simulink library "Airframes"  (Simulink 7.3)
settings: Solver=ode45  StartTime=0.0  StopTime=10.0  RelTol=1e-3
undefined symbols (not defined in the file or in its folder): Vo
libraries: aero_sim_lib x4, simulink x2
(part 1 of 2)
settings Model: Creator=Administrator  LastModifiedBy=Administrator

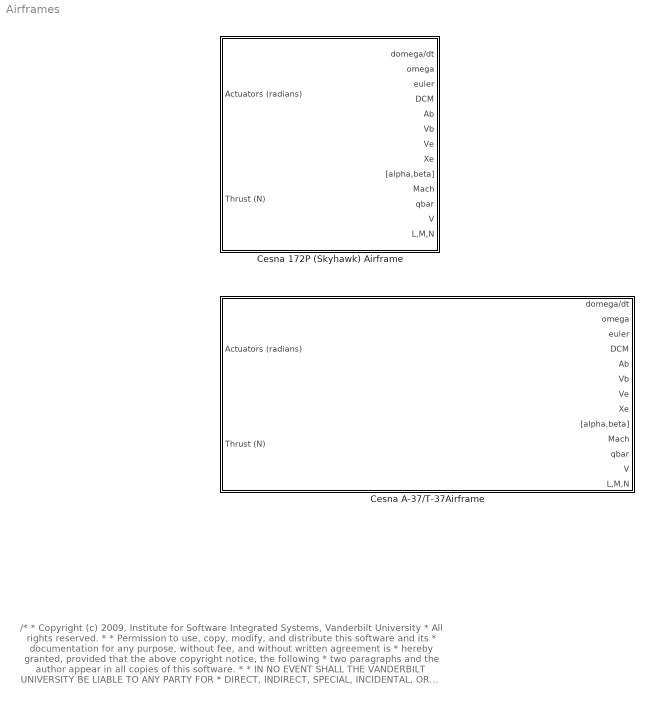
== system Airframes ==
  note: /*
      |  * Copyright (c) 2009, Institute for Software Integrated Systems, Vanderbilt University
      |  * All rights reserved.
      |  *
      |  * Permission to use, copy, modify, and distribute this software and its
      |  * documentation for any purpose, without fee, and without written agreement is
      |  * hereby granted, provided that the above copyright notice, the following
      |  * two paragraphs and the author appear in all copies of this software.
      |  *
      |  * IN NO EVENT SHALL THE VANDERBILT UNIVERSITY BE LIABLE TO ANY PARTY FOR
      |  * DIRECT, INDIRECT, SPECIAL, INCIDENTAL, OR CONSEQUENTIAL DAMAGES ARISING OUT
      |  * OF THE USE OF THIS SOFTWARE AND ITS DOCUMENTATION, EVEN IF THE VANDERBILT
      |  * UNIVERSITY HAS BEEN ADVISED OF THE POSSIBILITY OF SUCH DAMAGE.
      |  *
      |  * THE VANDERBILT UNIVERSITY SPECIFICALLY DISCLAIMS ANY WARRANTIES,
      |  * INCLUDING, BUT NOT LIMITED TO, THE IMPLIED WARRANTIES OF MERCHANTABILITY
      |  * AND FITNESS FOR A PARTICULAR PURPOSE.  THE SOFTWARE PROVIDED HEREUNDER IS
      |  * ON AN "AS IS" BASIS, AND THE VANDERBILT UNIVERSITY HAS NO OBLIGATION TO
      |  * PROVIDE MAINTENANCE, SUPPORT, UPDATES, ENHANCEMENTS, OR MODIFICATIONS.
      |  *
      |  * @author Nicholas Kottenstette
      |  */
  Cesna 172P (Skyhawk) Airframe : Subsystem  mask{trim_enable=off, XYZe_0=[0,0,-1000], V=Vo, Vb_0=Vo*[1,0,.0184], euler_0=[0,.018,0], omega_0=zeros(3,1), M=.4535959237*1043.3, I=[1285.3,0,0;0,1824.9,0;0,0,2666.9], b=10.9118, cbar=1.4935, S=16.1651, CG=[0,0,0], CP=[0,0,0], CD_p=[0.031,  0.13,  0,  0.06,  0], CL_p=[0.31,   5.143,    3.9,   0.43,   0], CY_p=[0,  -0.31,  -0.037,  0.21,  0.0,  0.187], Clm_p=[0, -0.089,  -0.47,  0.096,  -0.178,  0.0147], Cmm_p=[-0.015, -0.89,  -12.4,  -1.28,  0], Cnm_p=[0,  0.065, -0.03,  -0.099,  0.053,  -0.0657], delta_f=0, k_wind=off}
      mask prompts: trim_enable "Enable trim calculation"; XYZe_0 "Initial Inertial Position [XYZe_0] (meters)"; V "V (aero-velocity) (m/s)"; Vb_0 "Initial Body Velocity [Vb_0] (meters/sec)"; euler_0 "Initial Euler [euler_0] [roll,pitch,yaw] (radians)"; omega_0 "Initial Body Rotation Rates [omega_0] (rad/sec)"; M "Mass [M] (kg)"; I "Inertial Matrix [I] [Ixx,0,-Ixz;0,Iyy,0;-Ixz,0,Izz]"; b "Wing Span [b] (meters)"; cbar "MAC [cbar] (meters)"; S "Wing Area [S] (meters^2)"; CG "CG [CG] (meters)"; CP "CP [CP] (meters)"; CD_p "Drag Parameters:CD_p= [CD0,CDa,CDq,CDde,CDin]"; CL_p "Lift Parameters:CL_p=[CL0,CLa,CLq,CLde,CLin]"; CY_p "Y-Drag Parameters:CY_p=[CY0,CYb,CYp,CYr,CYda,CYdr]"; Clm_p "L-Moment (about-x_b) Parameters:Clm_p=[Cl0,Clb,Clp,Clr,Clda,Cldr]"; Cmm_p "M-Moment (about-y_b) Parameters:Cmm_p=[Cm0,Cma,Cmq,Cmde,Cmin]"; Cnm_p "N-Moment (about-z_b) Parameters:Cnm_p=[Cn0,Cnb,Cnp,Cnr,Cnda,Cndr]"; k_wind "wind dist on"
      mask init:
      | h=abs(XYZe_0(3));
      | if trim_enable
      |     [F_T_trim,alpha_trim,delta_e_trim,Sol] = fixed_wing_trim(CD_p,CL_p,Cmm_p,S,V,h,M,delta_f,[],false);
      |     u=V*sqrt(1/(1+tan(alpha_trim)^2));
      |     w=u*tan(alpha_trim);
      |     Vb_0=[u,0,w];
      |     euler_0(2)=alpha_trim;
      | end
      mask Display:
      | image(imread('Cessna_172P.jpg','jpg'))
      | color('black');port_label('output',1,'d\omega/dt','texmode','on')
      | port_label('output',2,'\omega','texmode','on')
      | port_label('output',3,'\eta^T=[\phi,\theta,\psi]^T','texmode','on')
      | port_label('output',4,'R(\eta)','texmode','on')
      | port_label('output',5,'A_b(m/s^2','texmode','on')
      | port_label('output',6,'V_b(m/s)','texmode','on')
      | port_label('output',7,'V_I(m/s)','texmode','on')
      | port_label('output',8,'X_I(m)','texmode','on')
      | port_label('output',9,'[\alpha,\beta]','texmode','on')
      | port_label('output',10,'Mach (V/a)')
      | port_label('output',11,'q_bar')
      | port_label('output',12,'V')
      | port_label('output',13,'L,M,N')
      | port_label('input',1,'[\delta_e,\delta_f,\delta_a,\delta_r](radians)','texmode','on')
      | port_label('input',2,'Thrust (N)')
  Cesna A-37/T-37Airframe : Subsystem  mask{trim_enable=off, XYZe_0=[0,0,-1000], V=Vo, Vb_0=Vo*[1,0,.0184], euler_0=[0,.018,0], omega_0=zeros(3,1), M=.4535959237*6360, I=1.35581795*[7.99e3,0,2.34e2;0,3.33e3,0;2.34e2,0,1.12e4], b=.3048*33.8, cbar=.3048*5.47, S=(.3048^2)*182, CG=[0,0,0], CP=[0,0,0], CD_p=[0.048,  0.384,  0,  0,  0], CL_p=[0.2,   5.15,    4.1,   0.5,   0], CY_p=[0,  -0.346,  -0.0827,  0.3,  0.0,  0.2], Clm_p=[0, -0.0944,  -0.442,  0.0926,  -0.181,  0.015], Cmm_p=[0.025, -0.7,  -14.9,  -1.12,  0], Cnm_p=[0,  0.1106, -0.0243,  -0.139,  0.0254,  -0.0365], delta_f=0, k_wind=off}
      mask prompts: trim_enable "Enable Trim Calculation"; XYZe_0 "Initial Inertial Position [XYZe_0] (meters)"; V "V (aero-velocity) (m/s)"; Vb_0 "Initial Body Velocity [Vb_0] (meters/sec)"; euler_0 "Initial Euler [euler_0] [roll,pitch,yaw] (radians)"; omega_0 "Initial Body Rotation Rates [omega_0] (rad/sec)"; M "Mass [M] (kg)"; I "Inertial Matrix [I] [Ixx,0,-Ixz;0,Iyy,0;-Ixz,0,Izz]"; b "Wing Span [b] (meters)"; cbar "MAC [cbar] (meters)"; S "Wing Area [S] (meters^2)"; CG "CG [CG] (meters)"; CP "CP [CP] (meters)"; CD_p "Drag Parameters:CD_p= [CD0,CDa,CDq,CDde,CDin]"; CL_p "Lift Parameters:CL_p=[CL0,CLa,CLq,CLde,CLin]"; CY_p "Y-Drag Parameters:CY_p=[CY0,CYb,CYp,CYr,CYda,CYdr]"; Clm_p "L-Moment (about-x_b) Parameters:Clm_p=[Cl0,Clb,Clp,Clr,Clda,Cldr]"; Cmm_p "M-Moment (about-y_b) Parameters:Cmm_p=[Cm0,Cma,Cmq,Cmde,Cmin]"; Cnm_p "N-Moment (about-z_b) Parameters:Cnm_p=[Cn0,Cnb,Cnp,Cnr,Cnda,Cndr]"; k_wind "wind dist on"
      mask init: same as Airframes/Cesna 172P (Skyhawk) Airframe
      mask Display:
      | image(imread('Cessna_T-37.jpg','jpg'))
      | color('magenta');port_label('output',1,'d\omega/dt','texmode','on')
      | port_label('output',2,'\omega','texmode','on')
      | port_label('output',3,'\eta^T=[\phi,\theta,\psi]^T','texmode','on')
      | port_label('output',4,'R(\eta)','texmode','on')
      | port_label('output',5,'A_b(m/s^2','texmode','on')
      | port_label('output',6,'V_b(m/s)','texmode','on')
      | port_label('output',7,'V_I(m/s)','texmode','on')
      | port_label('output',8,'X_I(m)','texmode','on')
      | port_label('output',9,'[\alpha,\beta]','texmode','on')
      | port_label('output',10,'Mach (V/a)')
      | port_label('output',11,'q_bar')
      | port_label('output',12,'V')
      | port_label('output',13,'L,M,N')
      | port_label('input',1,'[\delta_e,\delta_f,\delta_a,\delta_r](radians)','texmode','on')
      | port_label('input',2,'Thrust (N)')

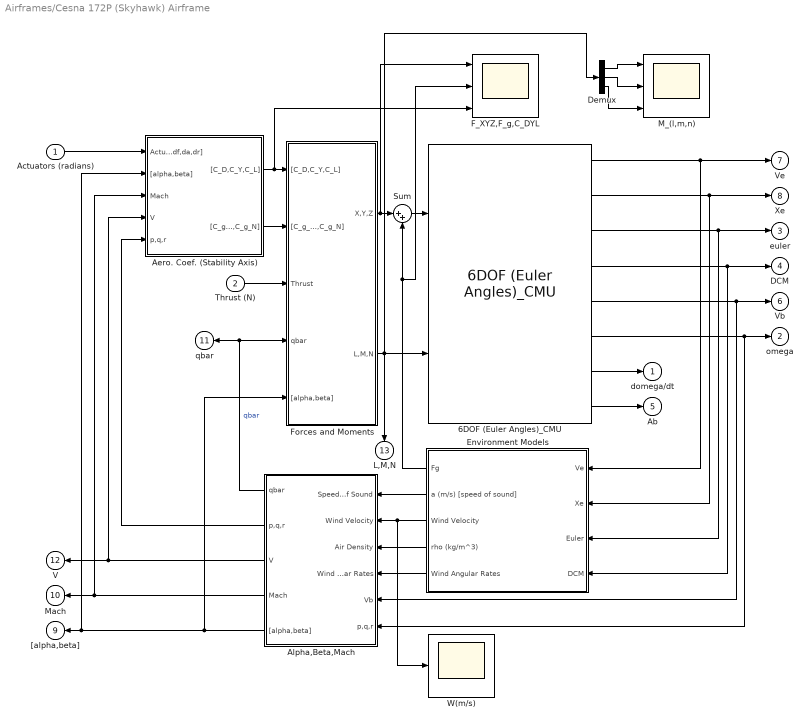
== system Airframes/Cesna 172P (Skyhawk) Airframe ==
  Actuators (radians) : Inport  OutDataType=sfix(16)  OutScaling=2^0
  Thrust (N) : Inport  Port=2  OutDataType=sfix(16)  OutScaling=2^0
  6DOF (Euler Angles)_CMU : aero_sim_lib/6DOF (Euler Angles)_CMU  SystemSampleTime=-1  XYZe_0=XYZe_0  Vb_0=Vb_0  euler_0=euler_0  omega_0=omega_0  M=M  I=I
  Aero. Coef. (Stability Axis) : Subsystem  mask{CD_p=CD_p, CL_p=CL_p, CY_p=CY_p, Clm_p=Clm_p, Cmm_p=Cmm_p, Cnm_p=Cnm_p, S=S, cbar=cbar, b=b}
      mask prompts: CD_p "Drag Parameters:CD_p= [CD0,CDa,CDq,CDde,CDin]"; CL_p "Lift Parameters:CL_p=[CL0,CLa,CLq,CLde,CLin]"; CY_p "Y-Drag Parameters:CY_p=[CY0,CYb,CYp,CYr,CYda,CYdr]"; Clm_p "L-Moment (about-x_b) Parameters:Clm_p=[Cl0,Clb,Clp,Clr,Clda,Cldr]"; Cmm_p "M-Moment (about-y_b) Parameters:Cmm_p=[Cm0,Cma,Cmq,Cmde,Cmin]"; Cnm_p "N-Moment (about-z_b) Parameters:Cnm_p=[Cn0,Cnb,Cnp,Cnr,Cnda,Cndr]"; S "Reference Area [S]"; cbar "MAC [cbar]"; b "wing span [b]"
  Alpha,Beta,Mach : Subsystem
  Demux : Demux  Outputs=3
  Environment Models : Subsystem
  F_XYZ,F_g,C_DYL : Scope  NumInputPorts=3
      settings: YMin=-5~-5~-5  YMax=5~5~5  SaveName=ScopeData3  SampleInput=on  SampleTime=0.01
  Forces and Moments : Subsystem
  M_(l,m,n) : Scope  NumInputPorts=3
      settings: YMin=-5~-5~-5  YMax=5~5~5  SaveName=ScopeData6  SampleInput=on  SampleTime=0.01
  Sum : Sum  Inputs=|++  OutDataType=sfix(16)  OutScaling=2^0  SaturateOnIntegerOverflow=on  InputSameDT=on  OutDataTypeStr=Inherit: Same as first input
  W(m/s) : Scope
      settings: YMin=-13  YMax=6  SaveName=ScopeData15  SampleInput=on  SampleTime=0.05
  domega/dt : Outport  OutDataType=sfix(16)  OutScaling=2^0  InitialOutput=0
  omega : Outport  Port=2  OutDataType=sfix(16)  OutScaling=2^0  InitialOutput=0
  euler : Outport  Port=3  OutDataType=sfix(16)  OutScaling=2^0  InitialOutput=0
  DCM : Outport  Port=4  OutDataType=sfix(16)  OutScaling=2^0  InitialOutput=0
  Ab : Outport  Port=5  OutDataType=sfix(16)  OutScaling=2^0  InitialOutput=0
  Vb : Outport  Port=6  OutDataType=sfix(16)  OutScaling=2^0  InitialOutput=0
  Ve : Outport  Port=7  OutDataType=sfix(16)  OutScaling=2^0  InitialOutput=0
  Xe : Outport  Port=8  OutDataType=sfix(16)  OutScaling=2^0  InitialOutput=0
  "[alpha,beta]" : Outport  Port=9  OutDataType=sfix(16)  OutScaling=2^0  InitialOutput=0
  Mach : Outport  Port=10  OutDataType=sfix(16)  OutScaling=2^0  InitialOutput=0
  qbar : Outport  Port=11  OutDataType=sfix(16)  OutScaling=2^0  InitialOutput=0
  V : Outport  Port=12  OutDataType=sfix(16)  OutScaling=2^0  InitialOutput=0
  L,M,N : Outport  Port=13  OutDataType=sfix(16)  OutScaling=2^0  InitialOutput=0
  wires:
  Aero. Coef. (Stability Axis)/2("[C_g_L,C_g_M,C_g_N]") -> Forces and Moments/2("[C_g_L,C_g_M,C_g_N]")
  6DOF (Euler Angles)_CMU/8 -> Ab/1
  6DOF (Euler Angles)_CMU/1 -> Environment Models/1(Ve), Ve/1
  6DOF (Euler Angles)_CMU/2 -> Environment Models/2(Xe), Xe/1
  6DOF (Euler Angles)_CMU/6 -> omega/1, Alpha,Beta,Mach/6(p,q,r)
  Thrust (N)/1 -> Forces and Moments/3(Thrust)
  6DOF (Euler Angles)_CMU/7 -> domega/dt/1
  6DOF (Euler Angles)_CMU/4 -> DCM/1, Environment Models/4(DCM)
  6DOF (Euler Angles)_CMU/3 -> Environment Models/3(Euler), euler/1
  Alpha,Beta,Mach/5("[alpha,beta]") -> Forces and Moments/5("[alpha,beta]"), "[alpha,beta]"/1, Aero. Coef. (Stability Axis)/2("[alpha,beta]")
  Aero. Coef. (Stability Axis)/1("[C_D,C_Y,C_L]") -> Forces and Moments/1("[C_D,C_Y,C_L]"), F_XYZ,F_g,C_DYL/3
  Environment Models/3(Wind Velocity) -> Alpha,Beta,Mach/2(Wind Velocity), W(m/s)/1
  6DOF (Euler Angles)_CMU/5 -> Alpha,Beta,Mach/5(Vb), Vb/1
  Environment Models/2(a (m/s) [speed of sound]) -> Alpha,Beta,Mach/1(Speed of Sound)
  Environment Models/4(rho (kg/m^3)) -> Alpha,Beta,Mach/3(Air Density)
  Forces and Moments/2(L,M,N) -> 6DOF (Euler Angles)_CMU/2, Demux/1, L,M,N/1
  Alpha,Beta,Mach/1(qbar) -> Forces and Moments/4(qbar), qbar/1  "qbar"
  Forces and Moments/1(X,Y,Z) -> Sum/1, F_XYZ,F_g,C_DYL/1
  Sum/1 -> 6DOF (Euler Angles)_CMU/1
  Environment Models/1(Fg) -> Sum/2, F_XYZ,F_g,C_DYL/2
  Actuators (radians)/1 -> Aero. Coef. (Stability Axis)/1(Actuators [de,df,da,dr])
  Alpha,Beta,Mach/3(V) -> Aero. Coef. (Stability Axis)/4(V), V/1
  Alpha,Beta,Mach/4(Mach) -> Aero. Coef. (Stability Axis)/3(Mach), Mach/1
  Alpha,Beta,Mach/2("p,q,r ") -> Aero. Coef. (Stability Axis)/5(p,q,r)
  Environment Models/5(Wind Angular Rates) -> Alpha,Beta,Mach/4(Wind Angular Rates)
  Demux/1 -> M_(l,m,n)/1
  Demux/2 -> M_(l,m,n)/2
  Demux/3 -> M_(l,m,n)/3

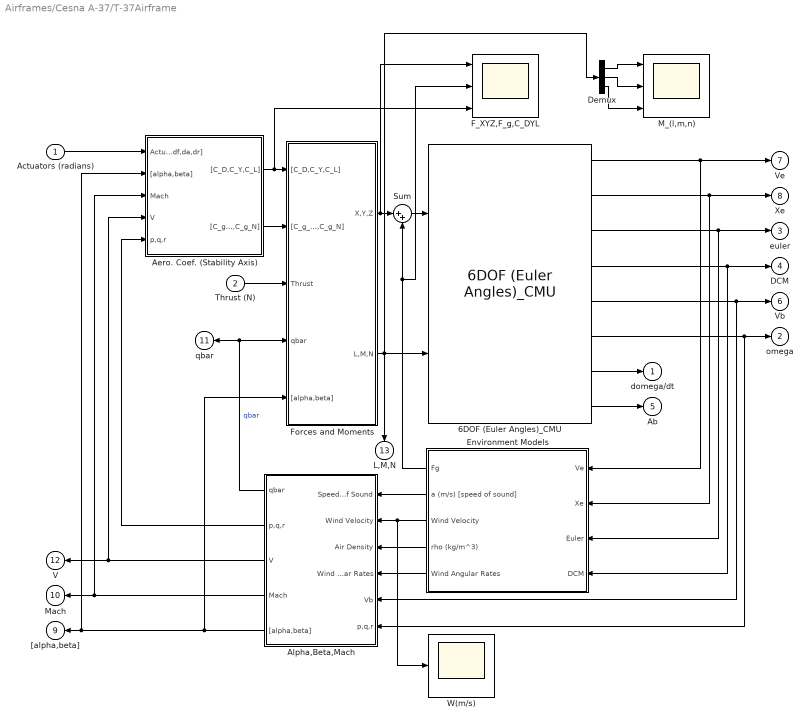
== system Airframes/Cesna A-37/T-37Airframe ==
  Actuators (radians) : Inport  OutDataType=sfix(16)  OutScaling=2^0
  Thrust (N) : Inport  Port=2  OutDataType=sfix(16)  OutScaling=2^0
  6DOF (Euler Angles)_CMU : aero_sim_lib/6DOF (Euler Angles)_CMU  SystemSampleTime=-1  XYZe_0=XYZe_0  Vb_0=Vb_0  euler_0=euler_0  omega_0=omega_0  M=M  I=I
  Aero. Coef. (Stability Axis) : Subsystem  mask{CD_p=CD_p, CL_p=CL_p, CY_p=CY_p, Clm_p=Clm_p, Cmm_p=Cmm_p, Cnm_p=Cnm_p, S=S, cbar=cbar, b=b}
      mask prompts: CD_p "Drag Parameters:CD_p= [CD0,CDa,CDq,CDde,CDin]"; CL_p "Lift Parameters:CL_p=[CL0,CLa,CLq,CLde,CLin]"; CY_p "Y-Drag Parameters:CY_p=[CY0,CYb,CYp,CYr,CYda,CYdr]"; Clm_p "L-Moment (about-x_b) Parameters:Clm_p=[Cl0,Clb,Clp,Clr,Clda,Cldr]"; Cmm_p "M-Moment (about-y_b) Parameters:Cmm_p=[Cm0,Cma,Cmq,Cmde,Cmin]"; Cnm_p "N-Moment (about-z_b) Parameters:Cnm_p=[Cn0,Cnb,Cnp,Cnr,Cnda,Cndr]"; S "Reference Area [S]"; cbar "MAC [cbar]"; b "wing span [b]"
  Alpha,Beta,Mach : Subsystem
  Demux : Demux  Outputs=3
  Environment Models : Subsystem
  F_XYZ,F_g,C_DYL : Scope  NumInputPorts=3
      settings: YMin=-5~-5~-5  YMax=5~5~5  SaveName=ScopeData3  SampleInput=on  SampleTime=0.01
  Forces and Moments : Subsystem
  M_(l,m,n) : Scope  NumInputPorts=3
      settings: YMin=-5~-5~-5  YMax=5~5~5  SaveName=ScopeData6  SampleInput=on  SampleTime=0.01
  Sum : Sum  Inputs=|++  OutDataType=sfix(16)  OutScaling=2^0  SaturateOnIntegerOverflow=on  InputSameDT=on  OutDataTypeStr=Inherit: Same as first input
  W(m/s) : Scope
      settings: YMin=-13  YMax=6  SaveName=ScopeData15  SampleInput=on  SampleTime=0.05
  domega/dt : Outport  OutDataType=sfix(16)  OutScaling=2^0  InitialOutput=0
  omega : Outport  Port=2  OutDataType=sfix(16)  OutScaling=2^0  InitialOutput=0
  euler : Outport  Port=3  OutDataType=sfix(16)  OutScaling=2^0  InitialOutput=0
  DCM : Outport  Port=4  OutDataType=sfix(16)  OutScaling=2^0  InitialOutput=0
  Ab : Outport  Port=5  OutDataType=sfix(16)  OutScaling=2^0  InitialOutput=0
  Vb : Outport  Port=6  OutDataType=sfix(16)  OutScaling=2^0  InitialOutput=0
  Ve : Outport  Port=7  OutDataType=sfix(16)  OutScaling=2^0  InitialOutput=0
  Xe : Outport  Port=8  OutDataType=sfix(16)  OutScaling=2^0  InitialOutput=0
  "[alpha,beta]" : Outport  Port=9  OutDataType=sfix(16)  OutScaling=2^0  InitialOutput=0
  Mach : Outport  Port=10  OutDataType=sfix(16)  OutScaling=2^0  InitialOutput=0
  qbar : Outport  Port=11  OutDataType=sfix(16)  OutScaling=2^0  InitialOutput=0
  V : Outport  Port=12  OutDataType=sfix(16)  OutScaling=2^0  InitialOutput=0
  L,M,N : Outport  Port=13  OutDataType=sfix(16)  OutScaling=2^0  InitialOutput=0
  wires:
  Demux/3 -> M_(l,m,n)/3
  Demux/2 -> M_(l,m,n)/2
  Demux/1 -> M_(l,m,n)/1
  Environment Models/5(Wind Angular Rates) -> Alpha,Beta,Mach/4(Wind Angular Rates)
  Alpha,Beta,Mach/2("p,q,r ") -> Aero. Coef. (Stability Axis)/5(p,q,r)
  Alpha,Beta,Mach/4(Mach) -> Mach/1, Aero. Coef. (Stability Axis)/3(Mach)
  Alpha,Beta,Mach/3(V) -> V/1, Aero. Coef. (Stability Axis)/4(V)
  Actuators (radians)/1 -> Aero. Coef. (Stability Axis)/1(Actuators [de,df,da,dr])
  Environment Models/1(Fg) -> F_XYZ,F_g,C_DYL/2, Sum/2
  Sum/1 -> 6DOF (Euler Angles)_CMU/1
  Forces and Moments/1(X,Y,Z) -> F_XYZ,F_g,C_DYL/1, Sum/1
  Alpha,Beta,Mach/1(qbar) -> qbar/1, Forces and Moments/4(qbar)  "qbar"
  Forces and Moments/2(L,M,N) -> L,M,N/1, Demux/1, 6DOF (Euler Angles)_CMU/2
  Environment Models/4(rho (kg/m^3)) -> Alpha,Beta,Mach/3(Air Density)
  Environment Models/2(a (m/s) [speed of sound]) -> Alpha,Beta,Mach/1(Speed of Sound)
  6DOF (Euler Angles)_CMU/5 -> Vb/1, Alpha,Beta,Mach/5(Vb)
  Environment Models/3(Wind Velocity) -> W(m/s)/1, Alpha,Beta,Mach/2(Wind Velocity)
  Aero. Coef. (Stability Axis)/1("[C_D,C_Y,C_L]") -> F_XYZ,F_g,C_DYL/3, Forces and Moments/1("[C_D,C_Y,C_L]")
  Alpha,Beta,Mach/5("[alpha,beta]") -> Aero. Coef. (Stability Axis)/2("[alpha,beta]"), "[alpha,beta]"/1, Forces and Moments/5("[alpha,beta]")
  6DOF (Euler Angles)_CMU/3 -> euler/1, Environment Models/3(Euler)
  6DOF (Euler Angles)_CMU/4 -> Environment Models/4(DCM), DCM/1
  6DOF (Euler Angles)_CMU/7 -> domega/dt/1
  Thrust (N)/1 -> Forces and Moments/3(Thrust)
  6DOF (Euler Angles)_CMU/6 -> Alpha,Beta,Mach/6(p,q,r), omega/1
  6DOF (Euler Angles)_CMU/2 -> Xe/1, Environment Models/2(Xe)
  6DOF (Euler Angles)_CMU/1 -> Ve/1, Environment Models/1(Ve)
  6DOF (Euler Angles)_CMU/8 -> Ab/1
  Aero. Coef. (Stability Axis)/2("[C_g_L,C_g_M,C_g_N]") -> Forces and Moments/2("[C_g_L,C_g_M,C_g_N]")

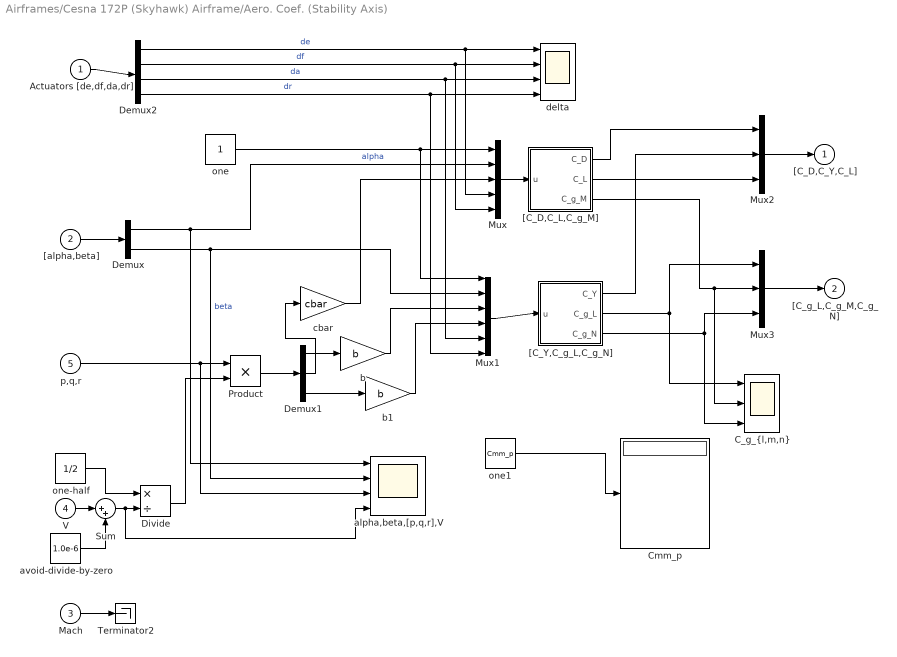
== system Airframes/Cesna 172P (Skyhawk) Airframe/Aero. Coef. (Stability Axis) ==
  Actuators [de,df,da,dr] : Inport  OutDataType=sfix(16)  OutScaling=2^0
  "[alpha,beta]" : Inport  Port=2  OutDataType=sfix(16)  OutScaling=2^0
  Mach : Inport  Port=3  OutDataType=sfix(16)  OutScaling=2^0
  V : Inport  Port=4  OutDataType=sfix(16)  OutScaling=2^0
  p,q,r : Inport  Port=5  OutDataType=sfix(16)  OutScaling=2^0
  "C_g_{l,m,n}" : Scope  NumInputPorts=3
      settings: YMin=-5~-5~-5  YMax=5~5~5  SaveName=ScopeData14  SampleInput=on  SampleTime=.01
  Cmm_p : Display
  Demux : Demux  Outputs=2
  Demux1 : Demux  Outputs=3
  Demux2 : Demux
  Divide : Product  Inputs=*/  OutDataType=fixdt(1, 16)  OutScaling=2^-10
  Mux : Mux  Inputs=5
  Mux1 : Mux  Inputs=6
  Mux2 : Mux  Inputs=3
  Mux3 : Mux  Inputs=3
  Product : Product  OutDataType=fixdt(1, 16)  OutScaling=2^0  RndMeth=Zero
  Sum : Sum  Inputs=|++  OutDataType=fixdt(1, 16)  OutScaling=2^0
  Terminator2 : Terminator
  "[C_D,C_L,C_g_M]" : Subsystem
  "[C_Y,C_g_L,C_g_N]" : Subsystem
  alpha,beta,[p,q,r],V : Scope  NumInputPorts=4
      settings: YMin=-5~-5~-5~-5  YMax=5~5~5~5  SaveName=ScopeData15  SampleInput=on  SampleTime=.01
  avoid-divide-by-zero : Constant  Value=1.0e-6  OutDataType=fixdt(1, 16)  OutScaling=2^0
  b : Gain  Gain=b  ParameterDataType=fixdt(1, 16)  ParameterScaling=2^0  OutDataType=fixdt(1, 16)  OutScaling=2^0
  b1 : Gain  Gain=b  ParameterDataType=fixdt(1, 16)  ParameterScaling=2^0  OutDataType=fixdt(1, 16)  OutScaling=2^0
  cbar : Gain  Gain=cbar  ParameterDataType=fixdt(1, 16)  ParameterScaling=2^0  OutDataType=fixdt(1, 16)  OutScaling=2^0
  delta : Scope  NumInputPorts=4
      settings: YMin=-5~-5~-5~-5  YMax=5~5~5~5  SaveName=ScopeData8  SampleInput=on  SampleTime=.01
  one : Constant  OutDataType=fixdt(1, 16)  OutScaling=2^0
  one-half : Constant  Value=1/2  OutDataType=fixdt(1, 16)  OutScaling=2^0
  one1 : Constant  Value=Cmm_p  OutDataType=fixdt(1, 16)  OutScaling=2^0
  "[C_D,C_Y,C_L]" : Outport  OutDataType=sfix(16)  OutScaling=2^0  InitialOutput=0
  "[C_g_L,C_g_M,C_g_N]" : Outport  Port=2  OutDataType=sfix(16)  OutScaling=2^0  InitialOutput=0
  wires:
  Mux3/1 -> "[C_g_L,C_g_M,C_g_N]"/1
  "[C_Y,C_g_L,C_g_N]"/3(C_g_N) -> Mux3/3, "C_g_{l,m,n}"/3
  "[C_Y,C_g_L,C_g_N]"/2(C_g_L) -> Mux3/1, "C_g_{l,m,n}"/1
  Mux2/1 -> "[C_D,C_Y,C_L]"/1
  "[C_Y,C_g_L,C_g_N]"/1(C_Y) -> Mux2/2
  Mux1/1 -> "[C_Y,C_g_L,C_g_N]"/1(u)
  Mux/1 -> "[C_D,C_L,C_g_M]"/1(u)
  "[C_D,C_L,C_g_M]"/3(C_g_M) -> Mux3/2, "C_g_{l,m,n}"/2
  "[C_D,C_L,C_g_M]"/2(C_L) -> Mux2/3
  "[C_D,C_L,C_g_M]"/1(C_D) -> Mux2/1
  Demux1/3 -> b1/1
  Demux1/1 -> b/1
  Demux/2 -> Mux1/2, alpha,beta,[p,q,r],V/2  "beta"
  Actuators [de,df,da,dr]/1 -> Demux2/1
  cbar/1 -> Mux/3
  Demux/1 -> Mux/2, alpha,beta,[p,q,r],V/1  "alpha"
  one/1 -> Mux1/1, Mux/1
  Product/1 -> Demux1/1
  Divide/1 -> Product/2
  p,q,r/1 -> Product/1, alpha,beta,[p,q,r],V/3
  avoid-divide-by-zero/1 -> Sum/2
  V/1 -> Sum/1
  Sum/1 -> Divide/2, alpha,beta,[p,q,r],V/4
  one-half/1 -> Divide/1
  "[alpha,beta]"/1 -> Demux/1
  Mach/1 -> Terminator2/1
  b/1 -> Mux1/3
  b1/1 -> Mux1/4
  Demux2/1 -> Mux/4, delta/1  "de"
  Demux2/2 -> Mux/5, delta/2  "df"
  Demux2/3 -> Mux1/5, delta/3  "da"
  Demux2/4 -> Mux1/6, delta/4  "dr"
  one1/1 -> Cmm_p/1
  Demux1/2 -> cbar/1

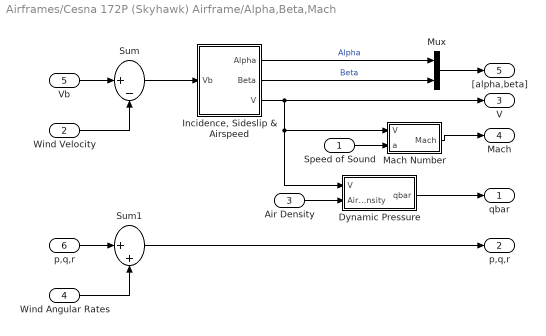
== system Airframes/Cesna 172P (Skyhawk) Airframe/Alpha,Beta,Mach ==
  Speed of Sound : Inport  OutDataType=sfix(16)  OutScaling=2^0
  Wind Velocity : Inport  Port=2  PortDimensions=3  OutDataType=sfix(16)  OutScaling=2^0
  Air Density : Inport  Port=3  OutDataType=sfix(16)  OutScaling=2^0
  Wind Angular Rates : Inport  Port=4  PortDimensions=3  OutDataType=sfix(16)  OutScaling=2^0
  Vb : Inport  Port=5  PortDimensions=3  OutDataType=sfix(16)  OutScaling=2^0
  p,q,r : Inport  Port=6  PortDimensions=3  OutDataType=sfix(16)  OutScaling=2^0
  Dynamic Pressure : Subsystem  mask(Dynamic Pressure){}
      mask help: Compute dynamic pressure using velocity and air density.
      mask init:
      | aeroicon('aeroblk');
      mask Help: eval('asbhelp');
      mask Display:
      | port_label('input',1,'V','texmode','on');
      | port_label('input',2,'\rho','texmode','on');
      | port_label('output',1,'q','texmode','on');
      | disp('^1/_2 \rhoV^2','texmode','on');
  "Incidence, Sideslip & Airspeed" : Subsystem  mask(Incidence,Sideslip,&Airspeed){}
      mask help: Calculate the angles between the body and the velocity vector (incidence and sideslip), and the velocity magnitude from the components in body axes (Vb).
      mask init:
      | aeroicon('aeroblk');
      mask Help: eval('asbhelp(''incidence_sideslip_and_airspeed'')');
      mask Display:
      | port_label('input',1,'V_b','texmode','on');
      | port_label('output',1,'\alpha','texmode','on');
      | port_label('output',2,'\beta','texmode','on');
      | port_label('output',3,'V','texmode','on');
  Mach Number : Subsystem  mask(Mach Number){}
      mask help: Compute Mach number using velocity and speed of sound.
      mask init:
      | aeroicon('aeroblk')
      mask Help: eval('asbhelp');
      mask Display:
      | port_label('input',1,'V','texmode','on');
      | port_label('input',2,'a','texmode','on');
      | port_label('output',1,'Mach','texmode','on');
  Mux : Mux  Inputs=2
  Sum : Sum  Inputs=|+-  OutDataType=sfix(16)  OutScaling=2^0  SaturateOnIntegerOverflow=on  InputSameDT=on  OutDataTypeStr=Inherit: Same as first input
  Sum1 : Sum  Inputs=|++  OutDataType=sfix(16)  OutScaling=2^0  SaturateOnIntegerOverflow=on  InputSameDT=on  OutDataTypeStr=Inherit: Same as first input
  qbar : Outport  OutDataType=sfix(16)  OutScaling=2^0  InitialOutput=0
  "p,q,r " : Outport  Port=2  OutDataType=sfix(16)  OutScaling=2^0
  V : Outport  Port=3  OutDataType=sfix(16)  OutScaling=2^0
  Mach : Outport  Port=4  OutDataType=sfix(16)  OutScaling=2^0
  "[alpha,beta]" : Outport  Port=5  OutDataType=sfix(16)  OutScaling=2^0
  wires:
  Mux/1 -> "[alpha,beta]"/1
  "Incidence, Sideslip & Airspeed"/3(V) -> Dynamic Pressure/1(V), Mach Number/1(V), V/1
  Dynamic Pressure/1(qbar) -> qbar/1
  Air Density/1 -> Dynamic Pressure/2(Air Density)
  Mach Number/1(Mach) -> Mach/1
  Sum/1 -> "Incidence, Sideslip & Airspeed"/1(Vb)
  Vb/1 -> Sum/1
  Speed of Sound/1 -> Mach Number/2(a)
  Wind Velocity/1 -> Sum/2
  "Incidence, Sideslip & Airspeed"/2(Beta) -> Mux/2  "Beta"
  "Incidence, Sideslip & Airspeed"/1(Alpha) -> Mux/1  "Alpha"
  p,q,r/1 -> Sum1/1
  Wind Angular Rates/1 -> Sum1/2
  Sum1/1 -> "p,q,r "/1

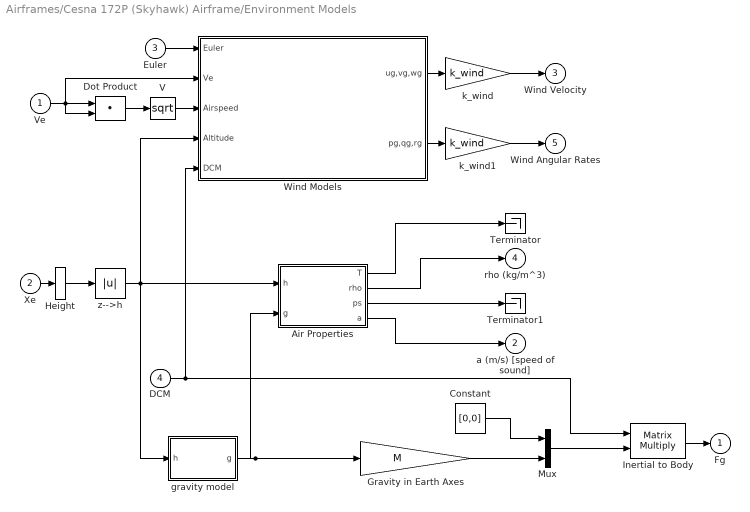
== system Airframes/Cesna 172P (Skyhawk) Airframe/Environment Models ==
  Ve : Inport  OutDataType=sfix(16)  OutScaling=2^0
  Xe : Inport  Port=2  PortDimensions=3  OutDataType=sfix(16)  OutScaling=2^0
  Euler : Inport  Port=3  OutDataType=sfix(16)  OutScaling=2^0
  DCM : Inport  Port=4  OutDataType=sfix(16)  OutScaling=2^0
  Air Properties : Stateflow chart
  Constant : Constant  Value=[0,0]  OutDataType=fixdt(1, 16)  OutScaling=2^0
  Dot Product : DotProduct  OutDataType=sfix(16)  OutScaling=2^-10  SaturateOnIntegerOverflow=on  OutDataTypeStr=Inherit: Inherit via internal rule
  Gravity in Earth Axes : Gain  Gain=M  ParameterDataType=sfix(16)  ParameterScaling=2^0  OutDataType=sfix(16)  OutScaling=2^0  SaturateOnIntegerOverflow=on  OutDataTypeStr=Inherit: Same as input  ParamDataTypeStr=Inherit: Same as input
  Height : Selector  InputPortWidth=3  IndexOptions=Index vector (dialog)  Indices=[3]  OutputSizes=1
  Inertial to Body : Product  Multiplication=Matrix(*)  OutDataType=sfix(16)  OutScaling=2^0  SaturateOnIntegerOverflow=on  InputSameDT=on  OutDataTypeStr=Inherit: Same as first input
  Mux : Mux  Inputs=[2,1]
  Terminator : Terminator
  Terminator1 : Terminator
  V : Math  Operator=sqrt  OutDataType=sfix(16)  OutScaling=2^0  SaturateOnIntegerOverflow=on
  Wind Models : Subsystem
  gravity model : Subsystem
  k_wind : Gain  Gain=k_wind  ParameterDataType=fixdt(1, 16)  ParameterScaling=2^0  OutDataType=fixdt(1, 16)  OutScaling=2^0
  k_wind1 : Gain  Gain=k_wind  ParameterDataType=fixdt(1, 16)  ParameterScaling=2^0  OutDataType=fixdt(1, 16)  OutScaling=2^0
  z-->h : Abs  SaturateOnIntegerOverflow=on
  Fg : Outport  OutDataType=sfix(16)  OutScaling=2^0  InitialOutput=0
  a (m/s) [speed of sound] : Outport  Port=2  OutDataType=sfix(16)  OutScaling=2^0  InitialOutput=0
  Wind Velocity : Outport  Port=3  OutDataType=sfix(16)  OutScaling=2^0  InitialOutput=0
  rho (kg/m^3) : Outport  Port=4  OutDataType=sfix(16)  OutScaling=2^0  InitialOutput=0
  Wind Angular Rates : Outport  Port=5  OutDataType=sfix(16)  OutScaling=2^0  InitialOutput=0
  wires:
  Constant/1 -> Mux/1
  Air Properties/3(ps) -> Terminator1/1
  Air Properties/4(a) -> a (m/s) [speed of sound]/1
  Air Properties/2(rho) -> rho (kg/m^3)/1
  Air Properties/1(T) -> Terminator/1
  Mux/1 -> Inertial to Body/2
  Euler/1 -> Wind Models/1(Euler)
  Ve/1 -> Wind Models/2(Ve), Dot Product/1, Dot Product/2
  Wind Models/1(ug,vg,wg) -> k_wind/1
  Wind Models/2(pg,qg,rg) -> k_wind1/1
  Dot Product/1 -> V/1
  z-->h/1 -> Air Properties/1(h), gravity model/1(h), Wind Models/4(Altitude)
  Height/1 -> z-->h/1
  Xe/1 -> Height/1
  gravity model/1(g) -> Air Properties/2(g), Gravity in Earth Axes/1
  Gravity in Earth Axes/1 -> Mux/2
  DCM/1 -> Wind Models/5(DCM), Inertial to Body/1
  Inertial to Body/1 -> Fg/1
  V/1 -> Wind Models/3(Airspeed)
  k_wind/1 -> Wind Velocity/1
  k_wind1/1 -> Wind Angular Rates/1

== system Airframes/Cesna 172P (Skyhawk) Airframe/Forces and Moments ==
  "[C_D,C_Y,C_L]" : Inport  OutDataType=sfix(16)  OutScaling=2^0
  "[C_g_L,C_g_M,C_g_N]" : Inport  Port=2  OutDataType=sfix(16)  OutScaling=2^0
  Thrust : Inport  Port=3  OutDataType=sfix(16)  OutScaling=2^0
  qbar : Inport  Port=4  OutDataType=sfix(16)  OutScaling=2^0
  "[alpha,beta]" : Inport  Port=5  OutDataType=sfix(16)  OutScaling=2^0
  Aero_Forces_Moments : Subsystem  mask{C_D_input_axes=Stability, C_g_L_input_axes=Body, S=S, b=b, cbar=cbar}
      mask prompts: C_D_input_axes "Drag Coef. Input Axes:"; C_g_L_input_axes "Moment Coef. Input Axes:"; S "Ref Area [S](m^2):"; b "Ref Span [b] (m):"; cbar "Ref Length [cbar] (m):"
      mask StyleString: popup(Stability|Wind|Body),popup(Stability|Wind|Body),edit,edit,edit
  CG : Constant  Value=CG  OutDataType=fixdt(1, 16)  OutScaling=2^0
  CP : Constant  Value=CP  OutDataType=fixdt(1, 16)  OutScaling=2^0
  Sum : Sum  Inputs=++|  OutDataType=sfix(16)  OutScaling=2^0  SaturateOnIntegerOverflow=on  InputSameDT=on  OutDataTypeStr=Inherit: Same as first input
  X,Y,Z : Outport  OutDataType=sfix(16)  OutScaling=2^0  InitialOutput=0
  L,M,N : Outport  Port=2  OutDataType=sfix(16)  OutScaling=2^0  InitialOutput=0
  wires:
  CP/1 -> Aero_Forces_Moments/6(CP)
  CG/1 -> Aero_Forces_Moments/5(CG)
  Aero_Forces_Moments/1(F_body) -> Sum/2
  Aero_Forces_Moments/2(M_body) -> L,M,N/1
  "[alpha,beta]"/1 -> Aero_Forces_Moments/1(alpha_beta)
  qbar/1 -> Aero_Forces_Moments/4(qbar)
  "[C_D,C_Y,C_L]"/1 -> Aero_Forces_Moments/2(C_DYL)
  "[C_g_L,C_g_M,C_g_N]"/1 -> Aero_Forces_Moments/3(C_g_LMN)
  Sum/1 -> X,Y,Z/1
  Thrust/1 -> Sum/1

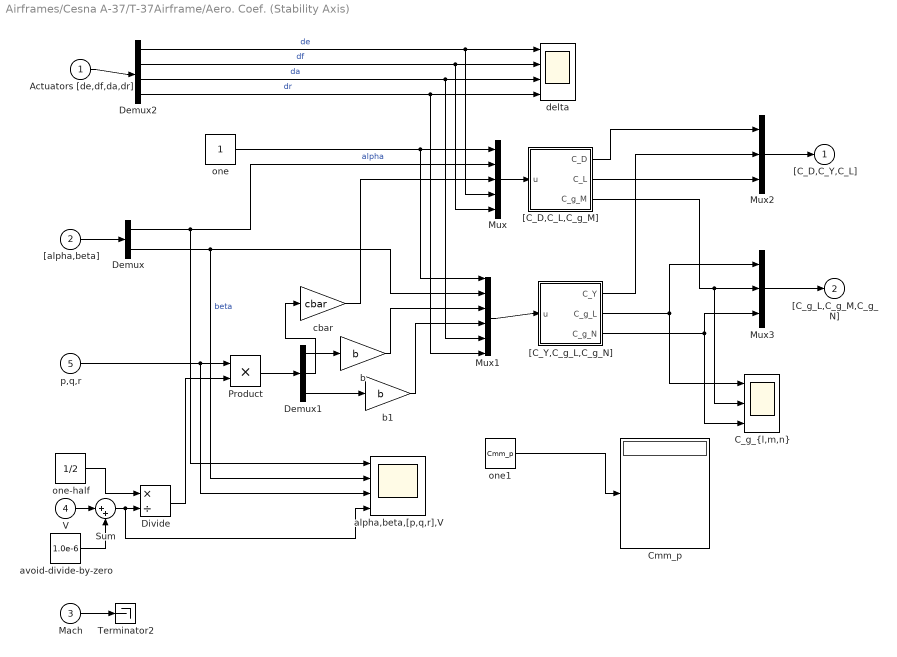
== system Airframes/Cesna A-37/T-37Airframe/Aero. Coef. (Stability Axis) ==
  Actuators [de,df,da,dr] : Inport  OutDataType=sfix(16)  OutScaling=2^0
  "[alpha,beta]" : Inport  Port=2  OutDataType=sfix(16)  OutScaling=2^0
  Mach : Inport  Port=3  OutDataType=sfix(16)  OutScaling=2^0
  V : Inport  Port=4  OutDataType=sfix(16)  OutScaling=2^0
  p,q,r : Inport  Port=5  OutDataType=sfix(16)  OutScaling=2^0
  "C_g_{l,m,n}" : Scope  NumInputPorts=3
      settings: YMin=-5~-5~-5  YMax=5~5~5  SaveName=ScopeData14  SampleInput=on  SampleTime=.01
  Cmm_p : Display
  Demux : Demux  Outputs=2
  Demux1 : Demux  Outputs=3
  Demux2 : Demux
  Divide : Product  Inputs=*/  OutDataType=fixdt(1, 16)  OutScaling=2^-10
  Mux : Mux  Inputs=5
  Mux1 : Mux  Inputs=6
  Mux2 : Mux  Inputs=3
  Mux3 : Mux  Inputs=3
  Product : Product  OutDataType=fixdt(1, 16)  OutScaling=2^0  RndMeth=Zero
  Sum : Sum  Inputs=|++  OutDataType=fixdt(1, 16)  OutScaling=2^0
  Terminator2 : Terminator
  "[C_D,C_L,C_g_M]" : Subsystem
  "[C_Y,C_g_L,C_g_N]" : Subsystem
  alpha,beta,[p,q,r],V : Scope  NumInputPorts=4
      settings: YMin=-5~-5~-5~-5  YMax=5~5~5~5  SaveName=ScopeData15  SampleInput=on  SampleTime=.01
  avoid-divide-by-zero : Constant  Value=1.0e-6  OutDataType=fixdt(1, 16)  OutScaling=2^0
  b : Gain  Gain=b  ParameterDataType=fixdt(1, 16)  ParameterScaling=2^0  OutDataType=fixdt(1, 16)  OutScaling=2^0
  b1 : Gain  Gain=b  ParameterDataType=fixdt(1, 16)  ParameterScaling=2^0  OutDataType=fixdt(1, 16)  OutScaling=2^0
  cbar : Gain  Gain=cbar  ParameterDataType=fixdt(1, 16)  ParameterScaling=2^0  OutDataType=fixdt(1, 16)  OutScaling=2^0
  delta : Scope  NumInputPorts=4
      settings: YMin=-5~-5~-5~-5  YMax=5~5~5~5  SaveName=ScopeData8  SampleInput=on  SampleTime=.01
  one : Constant  OutDataType=fixdt(1, 16)  OutScaling=2^0
  one-half : Constant  Value=1/2  OutDataType=fixdt(1, 16)  OutScaling=2^0
  one1 : Constant  Value=Cmm_p  OutDataType=fixdt(1, 16)  OutScaling=2^0
  "[C_D,C_Y,C_L]" : Outport  OutDataType=sfix(16)  OutScaling=2^0  InitialOutput=0
  "[C_g_L,C_g_M,C_g_N]" : Outport  Port=2  OutDataType=sfix(16)  OutScaling=2^0  InitialOutput=0
  wires:
  Demux1/2 -> cbar/1
  one1/1 -> Cmm_p/1
  Demux2/4 -> delta/4, Mux1/6  "dr"
  Demux2/3 -> delta/3, Mux1/5  "da"
  Demux2/2 -> delta/2, Mux/5  "df"
  Demux2/1 -> delta/1, Mux/4  "de"
  b1/1 -> Mux1/4
  b/1 -> Mux1/3
  Mach/1 -> Terminator2/1
  "[alpha,beta]"/1 -> Demux/1
  one-half/1 -> Divide/1
  Sum/1 -> alpha,beta,[p,q,r],V/4, Divide/2
  V/1 -> Sum/1
  avoid-divide-by-zero/1 -> Sum/2
  p,q,r/1 -> alpha,beta,[p,q,r],V/3, Product/1
  Divide/1 -> Product/2
  Product/1 -> Demux1/1
  one/1 -> Mux/1, Mux1/1
  Demux/1 -> alpha,beta,[p,q,r],V/1, Mux/2  "alpha"
  cbar/1 -> Mux/3
  Actuators [de,df,da,dr]/1 -> Demux2/1
  Demux/2 -> alpha,beta,[p,q,r],V/2, Mux1/2  "beta"
  Demux1/1 -> b/1
  Demux1/3 -> b1/1
  "[C_D,C_L,C_g_M]"/1(C_D) -> Mux2/1
  "[C_D,C_L,C_g_M]"/2(C_L) -> Mux2/3
  "[C_D,C_L,C_g_M]"/3(C_g_M) -> "C_g_{l,m,n}"/2, Mux3/2
  Mux/1 -> "[C_D,C_L,C_g_M]"/1(u)
  Mux1/1 -> "[C_Y,C_g_L,C_g_N]"/1(u)
  "[C_Y,C_g_L,C_g_N]"/1(C_Y) -> Mux2/2
  Mux2/1 -> "[C_D,C_Y,C_L]"/1
  "[C_Y,C_g_L,C_g_N]"/2(C_g_L) -> "C_g_{l,m,n}"/1, Mux3/1
  "[C_Y,C_g_L,C_g_N]"/3(C_g_N) -> "C_g_{l,m,n}"/3, Mux3/3
  Mux3/1 -> "[C_g_L,C_g_M,C_g_N]"/1

== system Airframes/Cesna A-37/T-37Airframe/Alpha,Beta,Mach ==
  Speed of Sound : Inport  OutDataType=sfix(16)  OutScaling=2^0
  Wind Velocity : Inport  Port=2  PortDimensions=3  OutDataType=sfix(16)  OutScaling=2^0
  Air Density : Inport  Port=3  OutDataType=sfix(16)  OutScaling=2^0
  Wind Angular Rates : Inport  Port=4  PortDimensions=3  OutDataType=sfix(16)  OutScaling=2^0
  Vb : Inport  Port=5  PortDimensions=3  OutDataType=sfix(16)  OutScaling=2^0
  p,q,r : Inport  Port=6  PortDimensions=3  OutDataType=sfix(16)  OutScaling=2^0
  Dynamic Pressure : Subsystem  mask(Dynamic Pressure){}
      mask help: Compute dynamic pressure using velocity and air density.
      mask init:
      | aeroicon('aeroblk');
      mask Help: eval('asbhelp');
      mask Display:
      | port_label('input',1,'V','texmode','on');
      | port_label('input',2,'\rho','texmode','on');
      | port_label('output',1,'q','texmode','on');
      | disp('^1/_2 \rhoV^2','texmode','on');
  "Incidence, Sideslip & Airspeed" : Subsystem  mask(Incidence,Sideslip,&Airspeed){}
      mask help: Calculate the angles between the body and the velocity vector (incidence and sideslip), and the velocity magnitude from the components in body axes (Vb).
      mask init:
      | aeroicon('aeroblk');
      mask Help: eval('asbhelp(''incidence_sideslip_and_airspeed'')');
      mask Display:
      | port_label('input',1,'V_b','texmode','on');
      | port_label('output',1,'\alpha','texmode','on');
      | port_label('output',2,'\beta','texmode','on');
      | port_label('output',3,'V','texmode','on');
  Mach Number : Subsystem  mask(Mach Number){}
      mask help: Compute Mach number using velocity and speed of sound.
      mask init:
      | aeroicon('aeroblk')
      mask Help: eval('asbhelp');
      mask Display:
      | port_label('input',1,'V','texmode','on');
      | port_label('input',2,'a','texmode','on');
      | port_label('output',1,'Mach','texmode','on');
  Mux : Mux  Inputs=2
  Sum : Sum  Inputs=|+-  OutDataType=sfix(16)  OutScaling=2^0  SaturateOnIntegerOverflow=on  InputSameDT=on  OutDataTypeStr=Inherit: Same as first input
  Sum1 : Sum  Inputs=|++  OutDataType=sfix(16)  OutScaling=2^0  SaturateOnIntegerOverflow=on  InputSameDT=on  OutDataTypeStr=Inherit: Same as first input
  qbar : Outport  OutDataType=sfix(16)  OutScaling=2^0  InitialOutput=0
  "p,q,r " : Outport  Port=2  OutDataType=sfix(16)  OutScaling=2^0
  V : Outport  Port=3  OutDataType=sfix(16)  OutScaling=2^0
  Mach : Outport  Port=4  OutDataType=sfix(16)  OutScaling=2^0
  "[alpha,beta]" : Outport  Port=5  OutDataType=sfix(16)  OutScaling=2^0
  wires:
  Sum1/1 -> "p,q,r "/1
  Wind Angular Rates/1 -> Sum1/2
  p,q,r/1 -> Sum1/1
  "Incidence, Sideslip & Airspeed"/1(Alpha) -> Mux/1  "Alpha"
  "Incidence, Sideslip & Airspeed"/2(Beta) -> Mux/2  "Beta"
  Wind Velocity/1 -> Sum/2
  Speed of Sound/1 -> Mach Number/2(a)
  Vb/1 -> Sum/1
  Sum/1 -> "Incidence, Sideslip & Airspeed"/1(Vb)
  Mach Number/1(Mach) -> Mach/1
  Air Density/1 -> Dynamic Pressure/2(Air Density)
  Dynamic Pressure/1(qbar) -> qbar/1
  "Incidence, Sideslip & Airspeed"/3(V) -> V/1, Mach Number/1(V), Dynamic Pressure/1(V)
  Mux/1 -> "[alpha,beta]"/1

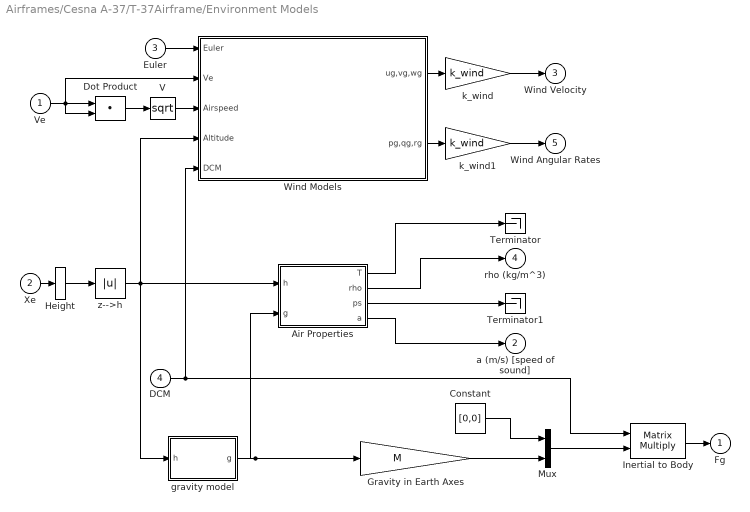
== system Airframes/Cesna A-37/T-37Airframe/Environment Models ==
  Ve : Inport  OutDataType=sfix(16)  OutScaling=2^0
  Xe : Inport  Port=2  PortDimensions=3  OutDataType=sfix(16)  OutScaling=2^0
  Euler : Inport  Port=3  OutDataType=sfix(16)  OutScaling=2^0
  DCM : Inport  Port=4  OutDataType=sfix(16)  OutScaling=2^0
  Air Properties : Stateflow chart
  Constant : Constant  Value=[0,0]  OutDataType=fixdt(1, 16)  OutScaling=2^0
  Dot Product : DotProduct  OutDataType=sfix(16)  OutScaling=2^-10  SaturateOnIntegerOverflow=on  OutDataTypeStr=Inherit: Inherit via internal rule
  Gravity in Earth Axes : Gain  Gain=M  ParameterDataType=sfix(16)  ParameterScaling=2^0  OutDataType=sfix(16)  OutScaling=2^0  SaturateOnIntegerOverflow=on  OutDataTypeStr=Inherit: Same as input  ParamDataTypeStr=Inherit: Same as input
  Height : Selector  InputPortWidth=3  IndexOptions=Index vector (dialog)  Indices=[3]  OutputSizes=1
  Inertial to Body : Product  Multiplication=Matrix(*)  OutDataType=sfix(16)  OutScaling=2^0  SaturateOnIntegerOverflow=on  InputSameDT=on  OutDataTypeStr=Inherit: Same as first input
  Mux : Mux  Inputs=[2,1]
  Terminator : Terminator
  Terminator1 : Terminator
  V : Math  Operator=sqrt  OutDataType=sfix(16)  OutScaling=2^0  SaturateOnIntegerOverflow=on
  Wind Models : Subsystem
  gravity model : Subsystem
  k_wind : Gain  Gain=k_wind  ParameterDataType=fixdt(1, 16)  ParameterScaling=2^0  OutDataType=fixdt(1, 16)  OutScaling=2^0
  k_wind1 : Gain  Gain=k_wind  ParameterDataType=fixdt(1, 16)  ParameterScaling=2^0  OutDataType=fixdt(1, 16)  OutScaling=2^0
  z-->h : Abs  SaturateOnIntegerOverflow=on
  Fg : Outport  OutDataType=sfix(16)  OutScaling=2^0  InitialOutput=0
  a (m/s) [speed of sound] : Outport  Port=2  OutDataType=sfix(16)  OutScaling=2^0  InitialOutput=0
  Wind Velocity : Outport  Port=3  OutDataType=sfix(16)  OutScaling=2^0  InitialOutput=0
  rho (kg/m^3) : Outport  Port=4  OutDataType=sfix(16)  OutScaling=2^0  InitialOutput=0
  Wind Angular Rates : Outport  Port=5  OutDataType=sfix(16)  OutScaling=2^0  InitialOutput=0
  wires:
  k_wind1/1 -> Wind Angular Rates/1
  k_wind/1 -> Wind Velocity/1
  V/1 -> Wind Models/3(Airspeed)
  Inertial to Body/1 -> Fg/1
  DCM/1 -> Inertial to Body/1, Wind Models/5(DCM)
  Gravity in Earth Axes/1 -> Mux/2
  gravity model/1(g) -> Gravity in Earth Axes/1, Air Properties/2(g)
  Xe/1 -> Height/1
  Height/1 -> z-->h/1
  z-->h/1 -> Wind Models/4(Altitude), gravity model/1(h), Air Properties/1(h)
  Dot Product/1 -> V/1
  Wind Models/2(pg,qg,rg) -> k_wind1/1
  Wind Models/1(ug,vg,wg) -> k_wind/1
  Ve/1 -> Dot Product/2, Dot Product/1, Wind Models/2(Ve)
  Euler/1 -> Wind Models/1(Euler)
  Mux/1 -> Inertial to Body/2
  Air Properties/1(T) -> Terminator/1
  Air Properties/2(rho) -> rho (kg/m^3)/1
  Air Properties/4(a) -> a (m/s) [speed of sound]/1
  Air Properties/3(ps) -> Terminator1/1
  Constant/1 -> Mux/1

== system Airframes/Cesna A-37/T-37Airframe/Forces and Moments ==
  "[C_D,C_Y,C_L]" : Inport  OutDataType=sfix(16)  OutScaling=2^0
  "[C_g_L,C_g_M,C_g_N]" : Inport  Port=2  OutDataType=sfix(16)  OutScaling=2^0
  Thrust : Inport  Port=3  OutDataType=sfix(16)  OutScaling=2^0
  qbar : Inport  Port=4  OutDataType=sfix(16)  OutScaling=2^0
  "[alpha,beta]" : Inport  Port=5  OutDataType=sfix(16)  OutScaling=2^0
  Aero_Forces_Moments : Subsystem  mask{C_D_input_axes=Stability, C_g_L_input_axes=Body, S=S, b=b, cbar=cbar}
      mask prompts: C_D_input_axes "Drag Coef. Input Axes:"; C_g_L_input_axes "Moment Coef. Input Axes:"; S "Ref Area [S](m^2):"; b "Ref Span [b] (m):"; cbar "Ref Length [cbar] (m):"
      mask StyleString: popup(Stability|Wind|Body),popup(Stability|Wind|Body),edit,edit,edit
  CG : Constant  Value=CG  OutDataType=fixdt(1, 16)  OutScaling=2^0
  CP : Constant  Value=CP  OutDataType=fixdt(1, 16)  OutScaling=2^0
  Sum : Sum  Inputs=++|  OutDataType=sfix(16)  OutScaling=2^0  SaturateOnIntegerOverflow=on  InputSameDT=on  OutDataTypeStr=Inherit: Same as first input
  X,Y,Z : Outport  OutDataType=sfix(16)  OutScaling=2^0  InitialOutput=0
  L,M,N : Outport  Port=2  OutDataType=sfix(16)  OutScaling=2^0  InitialOutput=0
  wires:
  Thrust/1 -> Sum/1
  Sum/1 -> X,Y,Z/1
  "[C_g_L,C_g_M,C_g_N]"/1 -> Aero_Forces_Moments/3(C_g_LMN)
  "[C_D,C_Y,C_L]"/1 -> Aero_Forces_Moments/2(C_DYL)
  qbar/1 -> Aero_Forces_Moments/4(qbar)
  "[alpha,beta]"/1 -> Aero_Forces_Moments/1(alpha_beta)
  Aero_Forces_Moments/2(M_body) -> L,M,N/1
  Aero_Forces_Moments/1(F_body) -> Sum/2
  CG/1 -> Aero_Forces_Moments/5(CG)
  CP/1 -> Aero_Forces_Moments/6(CP)

== system Airframes/Cesna 172P (Skyhawk) Airframe/Aero. Coef. (Stability Axis)/[C_D,C_L,C_g_M] ==
  u : Inport
  CD_p : Constant  Value=CD_p  OutDataType=fixdt(1, 16)  OutScaling=2^0
  CL_p : Constant  Value=CL_p  OutDataType=fixdt(1, 16)  OutScaling=2^0
  Cmm_p : Constant  Value=Cmm_p  OutDataType=fixdt(1, 16)  OutScaling=2^0
  Dot Product : DotProduct  OutDataType=fixdt(1, 16)  OutScaling=2^-10  InputSameDT=on  OutDataTypeStr=Inherit: Inherit via internal rule
  Dot Product1 : DotProduct  OutDataType=fixdt(1, 16)  OutScaling=2^-10  InputSameDT=on  OutDataTypeStr=Inherit: Inherit via internal rule
  Dot Product2 : DotProduct  OutDataType=fixdt(1, 16)  OutScaling=2^-10  InputSameDT=on  OutDataTypeStr=Inherit: Inherit via internal rule
  u1 : Display
  C_D : Outport
  C_L : Outport  Port=2
  C_g_M : Outport  Port=3
  wires:
  Dot Product2/1 -> C_g_M/1  "C_g_M"
  Dot Product1/1 -> C_L/1  "C_L"
  Dot Product/1 -> C_D/1  "C_D"
  Cmm_p/1 -> Dot Product2/2
  CD_p/1 -> Dot Product/2
  u/1 -> Dot Product/1, Dot Product1/1, Dot Product2/1, u1/1
  CL_p/1 -> Dot Product1/2

== system Airframes/Cesna 172P (Skyhawk) Airframe/Aero. Coef. (Stability Axis)/[C_Y,C_g_L,C_g_N] ==
  u : Inport
  CY_p : Constant  Value=CY_p  OutDataType=fixdt(1, 16)  OutScaling=2^0
  Clm_p : Constant  Value=Clm_p  OutDataType=fixdt(1, 16)  OutScaling=2^0
  Cmm_p : Constant  Value=Cnm_p  OutDataType=fixdt(1, 16)  OutScaling=2^0
  Dot Product : DotProduct  OutDataType=fixdt(1, 16)  OutScaling=2^-10  InputSameDT=on  OutDataTypeStr=Inherit: Inherit via internal rule
  Dot Product1 : DotProduct  OutDataType=fixdt(1, 16)  OutScaling=2^-10  InputSameDT=on  OutDataTypeStr=Inherit: Inherit via internal rule
  Dot Product2 : DotProduct  OutDataType=fixdt(1, 16)  OutScaling=2^-10  InputSameDT=on  OutDataTypeStr=Inherit: Inherit via internal rule
  C_Y : Outport
  C_g_L : Outport  Port=2
  C_g_N : Outport  Port=3
  wires:
  Clm_p/1 -> Dot Product1/2
  u/1 -> Dot Product2/1, Dot Product1/1, Dot Product/1
  CY_p/1 -> Dot Product/2
  Cmm_p/1 -> Dot Product2/2
  Dot Product/1 -> C_Y/1  "C_Y"
  Dot Product1/1 -> C_g_L/1  "C_g_L"
  Dot Product2/1 -> C_g_N/1  "C_g_N"

== system Airframes/Cesna 172P (Skyhawk) Airframe/Alpha,Beta,Mach/Dynamic Pressure ==
  V : Inport  OutDataType=sfix(16)  OutScaling=2^0
  Air Density : Inport  Port=2  OutDataType=sfix(16)  OutScaling=2^0
  1/2rhoV^2 : Gain  Gain=1/2  ParameterDataType=sfix(16)  ParameterScaling=2^0  OutDataType=sfix(16)  OutScaling=2^0  SaturateOnIntegerOverflow=on  OutDataTypeStr=Inherit: Same as input  ParamDataTypeStr=Inherit: Same as input
  Product1 : Product  OutDataType=sfix(16)  OutScaling=2^0  SaturateOnIntegerOverflow=on  InputSameDT=on  OutDataTypeStr=Inherit: Same as first input
  Product2 : Product  OutDataType=sfix(16)  OutScaling=2^0  SaturateOnIntegerOverflow=on  InputSameDT=on  OutDataTypeStr=Inherit: Same as first input
  qbar : Outport  OutDataType=sfix(16)  OutScaling=2^0  InitialOutput=0
  wires:
  V/1 -> Product1/2, Product1/1
  Product1/1 -> Product2/1
  Air Density/1 -> Product2/2
  Product2/1 -> 1/2rhoV^2/1
  1/2rhoV^2/1 -> qbar/1

== system Airframes/Cesna 172P (Skyhawk) Airframe/Alpha,Beta,Mach/Incidence, Sideslip & Airspeed ==
  Vb : Inport  OutDataType=sfix(16)  OutScaling=2^0
  Airspeed : Math  Operator=sqrt  OutDataType=sfix(16)  OutScaling=2^0  SaturateOnIntegerOverflow=on
  Dot Product : DotProduct  OutDataType=fixdt(1, 16)  OutScaling=2^-10  InputSameDT=on  OutDataTypeStr=Inherit: Inherit via internal rule
  Incidence : Trigonometry  Operator=atan2
  Product : Product  Inputs=*/  OutDataType=sfix(16)  OutScaling=2^0  SaturateOnIntegerOverflow=on  OutDataTypeStr=Inherit: Same as first input
  Sideslip : Trigonometry  Operator=asin
  Subsystem : Subsystem
  Subsystem1 : Subsystem
  Alpha : Outport  OutDataType=sfix(16)  OutScaling=2^0  InitialOutput=0
  Beta : Outport  Port=2  OutDataType=sfix(16)  OutScaling=2^0  InitialOutput=0
  V : Outport  Port=3  OutDataType=sfix(16)  OutScaling=2^0  InitialOutput=0
  wires:
  Subsystem1/1(v) -> Product/1
  Sideslip/1 -> Beta/1
  Vb/1 -> Dot Product/2, Dot Product/1, Subsystem1/1(Vb), Subsystem/1(Vb)
  Incidence/1 -> Alpha/1
  Airspeed/1 -> V/1, Product/2
  Dot Product/1 -> Airspeed/1
  Subsystem/2(u) -> Incidence/2
  Subsystem/1(w) -> Incidence/1
  Product/1 -> Sideslip/1

== system Airframes/Cesna 172P (Skyhawk) Airframe/Alpha,Beta,Mach/Mach Number ==
  V : Inport  OutDataType=sfix(16)  OutScaling=2^0
  a : Inport  Port=2  OutDataType=sfix(16)  OutScaling=2^0
  Product1 : Product  Inputs=*/  OutDataType=sfix(16)  OutScaling=2^0  SaturateOnIntegerOverflow=on  InputSameDT=on  OutDataTypeStr=Inherit: Same as first input
  Mach : Outport  OutDataType=sfix(16)  OutScaling=2^0
  wires:
  V/1 -> Product1/1
  a/1 -> Product1/2
  Product1/1 -> Mach/1

== system Airframes/Cesna 172P (Skyhawk) Airframe/Environment Models/Wind Models ==
  Euler : Inport  OutDataType=sfix(16)  OutScaling=2^0
  Ve : Inport  Port=2  OutDataType=sfix(16)  OutScaling=2^0
  Airspeed : Inport  Port=3  OutDataType=sfix(16)  OutScaling=2^0
  Altitude : Inport  Port=4  OutDataType=sfix(16)  OutScaling=2^0
  DCM : Inport  Port=5  OutDataType=sfix(16)  OutScaling=2^0
  MIL-F-8785C Wind Gust Model (to do) : Subsystem  mask{G_u=on, G_v=on, G_w=on, t_0=100, x_m=10*[b,b,b], v_m=[5,5,5]}
      mask prompts: G_u "Gust in u-axis [G_u]"; G_v "Gust in v-axis [G_v]"; G_w "Gust in w-axis [G_w]"; t_0 "Gust start-time [t_0] (sec):"; x_m "Gust legth x_m=[x_u,x_v,x_w] (m):"; v_m "Gust amplitude v_m=[v_u,v_v,v_w](m/s):"
  MIL-F-8785C Wind Shear Model : Subsystem  mask{phase=Category C (Terminal Flight), u20=6, deg=0}
      mask prompts: phase "Select Flight Phase [phase]"; u20 "Wind Speed at 20 feet above ground [u20] (m/sec)"; deg "Approach Angle of Wind (clock-wise from the North) [deg] (degrees)"
      mask StyleString: popup(Category C (Terminal Flight)|Category A or B (Not Terminal Flight)),edit,edit
  Need Dryden Turbulent Model Block : Constant  Value=[0,0,0]  OutDataType=fixdt(1, 16)  OutScaling=2^0
  Sum : Sum  Inputs=+|+  OutDataType=sfix(16)  OutScaling=2^0  SaturateOnIntegerOverflow=on  InputSameDT=on  OutDataTypeStr=Inherit: Same as first input
  Terminator : Terminator
  Terminator1 : Terminator
  ug,vg,wg : Outport  OutDataType=sfix(16)  OutScaling=2^0
  pg,qg,rg : Outport  Port=2  OutDataType=sfix(16)  OutScaling=2^0
  wires:
  Need Dryden Turbulent Model Block/1 -> pg,qg,rg/1
  MIL-F-8785C Wind Gust Model (to do)/1(v_w(m/s)) -> Sum/2
  MIL-F-8785C Wind Shear Model/1(v_w) -> Sum/1
  Euler/1 -> Terminator1/1
  Ve/1 -> Terminator/1
  Sum/1 -> ug,vg,wg/1
  DCM/1 -> MIL-F-8785C Wind Shear Model/2(DCM)
  Airspeed/1 -> MIL-F-8785C Wind Gust Model (to do)/1(V(m/s))
  Altitude/1 -> MIL-F-8785C Wind Shear Model/1(h)

== system Airframes/Cesna 172P (Skyhawk) Airframe/Environment Models/gravity model ==
  h : Inport
  Divide : Product  Inputs=*/  OutDataType=fixdt(1, 16)  OutScaling=2^-10
  Dot Product1 : DotProduct  OutDataType=fixdt(1, 16)  OutScaling=2^-10  InputSameDT=on  OutDataTypeStr=Inherit: Inherit via internal rule
  Model Info : simulink/Model-Wide Utilities/Model Info  SystemSampleTime=-1  InitialBlockCM=None  BlockCM=None  Frame=on  DisplayStringWithTags=g = g_o [R/(R+h)]^2  HorizontalTextAlignment=Center  LeftAlignmentValue=0.5  SourceBlockDiagram=Airframes  TagMaxNumber=20
  R = Radius of Earth (m) : Constant  Value=6356e3  OutDataType=fixdt(1, 16)  OutScaling=2^0
  Sum : Sum  Inputs=|++  OutDataType=fixdt(1, 16)  OutScaling=2^0
  g_o : Gain  Gain=9.80665  ParameterDataType=fixdt(1, 16)  ParameterScaling=2^0  OutDataType=fixdt(1, 16)  OutScaling=2^0
  g : Outport
  wires:
  g_o/1 -> g/1
  h/1 -> Sum/1
  Dot Product1/1 -> g_o/1
  Divide/1 -> Dot Product1/2, Dot Product1/1
  Sum/1 -> Divide/2
  R = Radius of Earth (m)/1 -> Divide/1, Sum/2

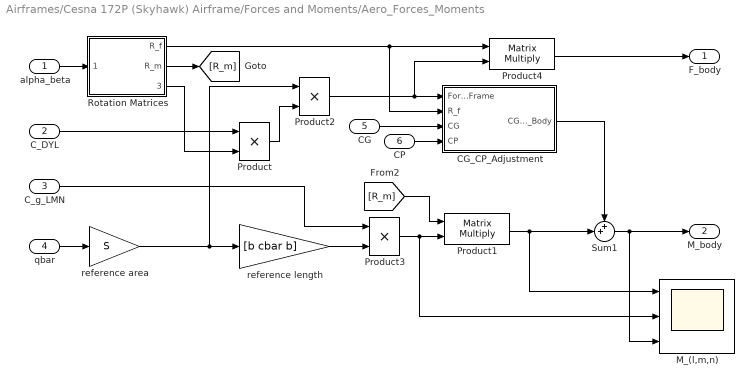
== system Airframes/Cesna 172P (Skyhawk) Airframe/Forces and Moments/Aero_Forces_Moments ==
  alpha_beta : Inport
  C_DYL : Inport  Port=2
  C_g_LMN : Inport  Port=3
  qbar : Inport  Port=4
  CG : Inport  Port=5  OutDataType=sfix(16)  OutScaling=2^0
  CP : Inport  Port=6  OutDataType=sfix(16)  OutScaling=2^0
  CG_CP_Adjustment : Subsystem
  M_(l,m,n) : Scope  NumInputPorts=3
      settings: YMin=-5~-5~-5  YMax=5~5~5  SaveName=ScopeData7  SampleInput=on  SampleTime=0.01
  Product : Product  OutDataType=sfix(16)  OutScaling=2^0  SaturateOnIntegerOverflow=on  InputSameDT=on  OutDataTypeStr=Inherit: Same as first input
  Product1 : Product  Multiplication=Matrix(*)  OutDataType=sfix(16)  OutScaling=2^0  RndMeth=Zero
  Product2 : Product  OutDataType=sfix(16)  OutScaling=2^0  SaturateOnIntegerOverflow=on  InputSameDT=on  OutDataTypeStr=Inherit: Same as first input
  Product3 : Product  OutDataType=sfix(16)  OutScaling=2^0  SaturateOnIntegerOverflow=on  InputSameDT=on  OutDataTypeStr=Inherit: Same as first input
  Product4 : Product  Multiplication=Matrix(*)  OutDataType=sfix(16)  OutScaling=2^0  RndMeth=Zero
  Rotation Matrices : Stateflow chart
  Sum1 : Sum  Inputs=++|  OutDataType=sfix(16)  OutScaling=2^0  SaturateOnIntegerOverflow=on  InputSameDT=on  OutDataTypeStr=Inherit: Same as first input
  reference area : Gain  Gain=S  ParameterDataType=sfix(16)  ParameterScaling=2^0  OutDataType=sfix(16)  OutScaling=2^0  SaturateOnIntegerOverflow=on  OutDataTypeStr=Inherit: Same as input  ParamDataTypeStr=Inherit: Same as input
  reference length : Gain  Gain=[b cbar b]  ParameterDataType=sfix(16)  ParameterScaling=2^0  OutDataType=sfix(16)  OutScaling=2^0  SaturateOnIntegerOverflow=on  OutDataTypeStr=Inherit: Same as input  ParamDataTypeStr=Inherit: Same as input
  F_body : Outport
  M_body : Outport  Port=2
  wires:
  Sum1/1 -> M_body/1, M_(l,m,n)/3
  CG_CP_Adjustment/1(CGP_M_Body) -> Sum1/1
  Product1/1 -> Sum1/2, M_(l,m,n)/1
  Product3/1 -> Product1/2, M_(l,m,n)/2
  [R_m] -> Product1/1
  Rotation Matrices/2(R_m) -> [R_m]
  Product4/1 -> F_body/1
  Product2/1 -> CG_CP_Adjustment/1(Forces_Drag_Frame), Product4/2
  Product/1 -> Product2/2
  Rotation Matrices/1(R_f) -> CG_CP_Adjustment/2(R_f), Product4/1
  CP/1 -> CG_CP_Adjustment/4(CP)
  CG/1 -> CG_CP_Adjustment/3(CG)
  C_g_LMN/1 -> Product3/1
  reference length/1 -> Product3/2
  Rotation Matrices/3(K_adjust) -> Product/2
  C_DYL/1 -> Product/1
  reference area/1 -> Product2/1, reference length/1
  qbar/1 -> reference area/1
  alpha_beta/1 -> Rotation Matrices/1(alpha_beta)

== system Airframes/Cesna A-37/T-37Airframe/Aero. Coef. (Stability Axis)/[C_D,C_L,C_g_M] ==
  u : Inport
  CD_p : Constant  Value=CD_p  OutDataType=fixdt(1, 16)  OutScaling=2^0
  CL_p : Constant  Value=CL_p  OutDataType=fixdt(1, 16)  OutScaling=2^0
  Cmm_p : Constant  Value=Cmm_p  OutDataType=fixdt(1, 16)  OutScaling=2^0
  Dot Product : DotProduct  OutDataType=fixdt(1, 16)  OutScaling=2^-10  InputSameDT=on  OutDataTypeStr=Inherit: Inherit via internal rule
  Dot Product1 : DotProduct  OutDataType=fixdt(1, 16)  OutScaling=2^-10  InputSameDT=on  OutDataTypeStr=Inherit: Inherit via internal rule
  Dot Product2 : DotProduct  OutDataType=fixdt(1, 16)  OutScaling=2^-10  InputSameDT=on  OutDataTypeStr=Inherit: Inherit via internal rule
  u1 : Display
  C_D : Outport
  C_L : Outport  Port=2
  C_g_M : Outport  Port=3
  wires:
  CL_p/1 -> Dot Product1/2
  u/1 -> u1/1, Dot Product2/1, Dot Product1/1, Dot Product/1
  CD_p/1 -> Dot Product/2
  Cmm_p/1 -> Dot Product2/2
  Dot Product/1 -> C_D/1  "C_D"
  Dot Product1/1 -> C_L/1  "C_L"
  Dot Product2/1 -> C_g_M/1  "C_g_M"
